simulink subsystem "brakeBias"  (R2022b)
settings: Solver=VariableStepAuto  StartTime=0.0  StopTime=10.0  RelTol=1e-3
libraries: brake_lib x1, Raptor_lib x1
settings Model: Creator=serga  LastModifiedBy=serga

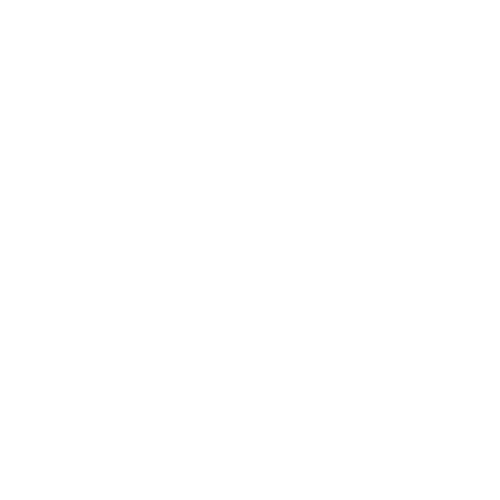
[thumbnail: Simulink's stored preview of the top-level diagram]
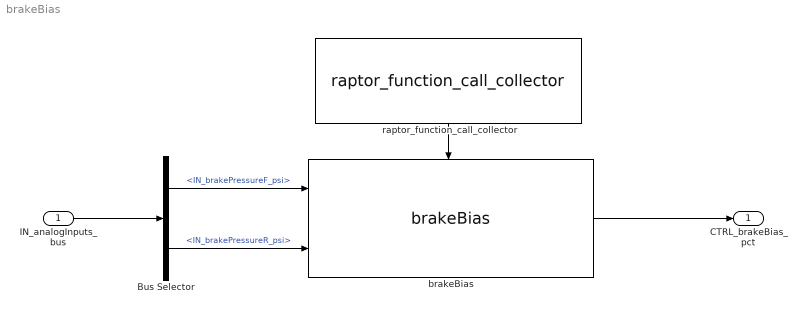
== system brakeBias ==
  IN_analogInputs_bus : Inport
  Bus Selector : BusSelector  OutputSignals=IN_brake_bus.IN_brakeF_bus.IN_brakePressureF_psi,IN_brake_bus.IN_brakeR_bus.IN_brakePressureR_psi
  brakeBias : brake_lib/brakeBias  SystemSampleTime=-1  VariantActivationTime=update diagram  Latency=0  AutoFrameSizeCalculation=off
  raptor_function_call_collector : Raptor_lib/Triggers/raptor_function_call_collector  count=5
      settings: SourceProductName=Raptor
  CTRL_brakeBias_pct : Outport
  wires:
  IN_analogInputs_bus/1 -> Bus Selector/1
  Bus Selector/1 -> brakeBias/1  "<IN_brakePressureF_psi>"
  Bus Selector/2 -> brakeBias/2  "<IN_brakePressureR_psi>"
  raptor_function_call_collector/1 -> brakeBias/Trigger
  brakeBias/1 -> CTRL_brakeBias_pct/1
